simulink model "house35"  (R2022b)
settings: Solver=VariableStepAuto  StartTime=0.0  StopTime=60  RelTol=1e-3
libraries: vrlib x1
settings Model: NumberOfSteps=5  Creator=Abdiladif Hassan  LastModifiedBy=Administrator
settings OptimizationCC: ReuseModelBlockBuffer=on

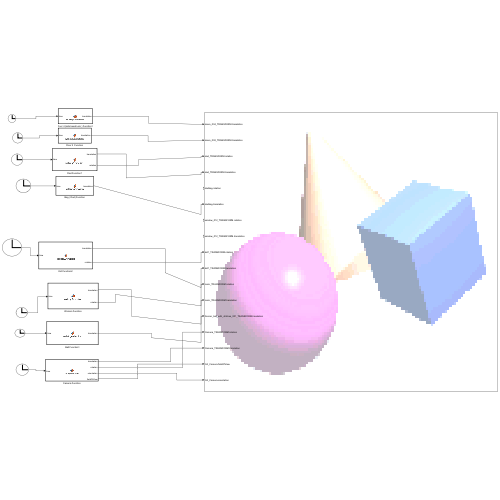
[thumbnail: Simulink's stored preview of the top-level diagram]
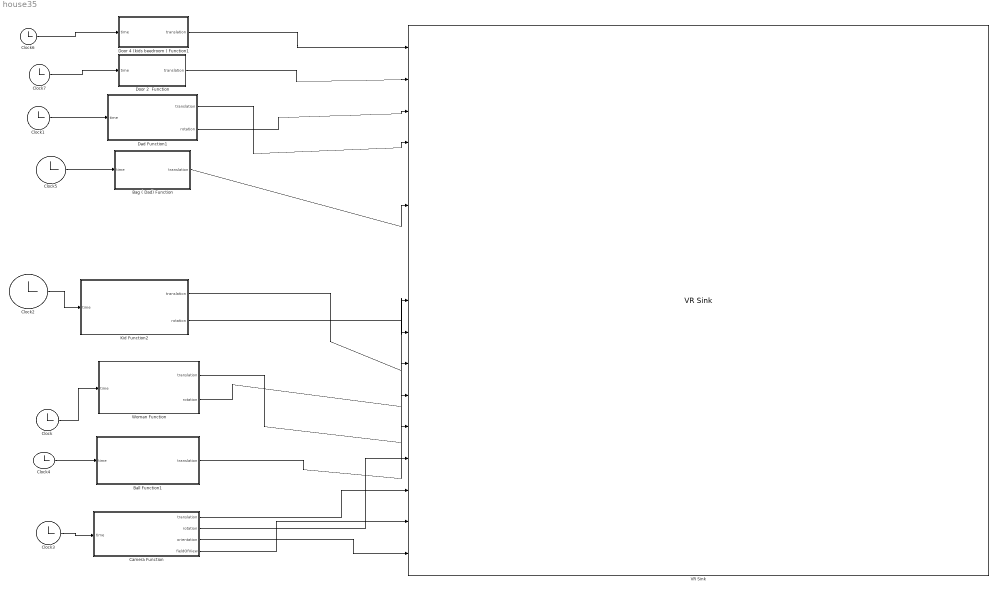
== system house35 ==
  Bag ( Dad) Function : MATLAB Function  TreatAsAtomicUnit=on
  Ball Function1 : MATLAB Function  TreatAsAtomicUnit=on
  Camera Function : MATLAB Function  TreatAsAtomicUnit=on
  Clock{,1..7} (8 alike) : Clock
  Dad Function1 : MATLAB Function  TreatAsAtomicUnit=on
  Door 2  Function : MATLAB Function  TreatAsAtomicUnit=on
  Door 4 (kids beedroom ) Function1 : MATLAB Function  TreatAsAtomicUnit=on
  Kid Function2 : MATLAB Function  TreatAsAtomicUnit=on
  VR Sink : vrlib/VR Sink  InstantiateOnLoad=on  SampleTime=0.1  ViewEnable=on  RemoteChange=off  RemoteView=off  FieldsWritten=dvere_004_TRANSFORM.translation.3.1.1.double#dvere_002_TRANSFORM.translation.3.1.1.double#dad_TRANSFORM.rotation.4.1.1.double#dad_TRANSFORM.translation.3.1.1.double#dadbag.rotation.4.1.1.double#dadbag.translation.3.1.1.double#window_012_TRANSFORM.rotation.4.1.1.double#window_012_TRANSFORM.translation.3.1.1.double#kid1_TRANSFORM.rotation.4.1.1.double#kid1_TRANSFORM.translation.3.1.1.double#mom_TRANSFORM.rotation.4.1.1.double#mom_TRANSFORM.translation.3.1.1.double#Soccer_ball_with_stitches_001_TRANSFORM.translation.3.1.1.double#Camera_TRANSFORM.rotation.4.1.1.double#Camera_TRANSFORM.translation.3.1.1.double#CA_Camera.fieldOfView.1.1.1.double#CA_Camera.orientation.4.1.1.double  WorldFileName=house35.x3d  AutoView=off  VideoDimensions=[]  AllowVariableSize=off  FigureProperties="{'Position', 'Name', 'Viewpoint', 'CameraBound', 'CameraDirection', 'CameraPosition', 'CameraUpVector', 'ZoomFactor', 'Antialiasing', 'Headlight', 'Lighting', 'NavPanel', 'Sound', 'StatusBar', 'Stereo3D', 'Stereo3DCameraOffset', 'Stereo3DHIT', 'ToolBar', 'Textures', 'Transparency', 'Triad', 'Wireframe', 'NavZones', 'NavMode', 'NavSpeed', 'CaptureFileFormat', 'CaptureFileName', 'Record2DCompressMethod', 'Record2DCompressQuality', 'Record2D', 'Record2DFileName', 'Record2DFPS'; [1.0000000000000000e+00   7.6000000000000000e+01   1.3660000000000000e+03   5.9300000000000000e+02], '', '_untitled_1', 'on', [0.0000000000000000e+00   0.0000000000000000e+00  -1.0000000000000000e+00], [0.0000000000000000e+00   0.0000000000000000e+00   0.0000000000000000e+00], [0.0000000000000000e+00   1.0000000000000000e+00   0.0000000000000000e+00], [1.0000000000000000e+00], 'on', 'on', 'on', 'halfbar', 'on', 'on', 'off', [1.0000000149011612e-01], [0.0000000000000000e+00], 'on', 'on', 'on', 'none', 'off', 'off', 'examine', 'normal', 'tif', 'C:\\Users\\Administrator\\Videos\\%f_anim_%n.tif', 'auto', [7.5000000000000000e+01], 'on', 'C:\\Users\\Administrator\\Videos\\%f_anim_%n.avi', 'auto'}"
  Woman Function : MATLAB Function  TreatAsAtomicUnit=on
  wires:
  Clock/1 -> Woman Function/1(time)
  Clock1/1 -> Dad Function1/1(time)
  Clock2/1 -> Kid Function2/1(time)
  Clock3/1 -> Camera Function/1(time)
  Clock4/1 -> Ball Function1/1(time)
  Clock5/1 -> Bag ( Dad) Function/1(time)
  Clock7/1 -> Door 2  Function/1(time)
  Clock6/1 -> Door 4 (kids beedroom ) Function1/1(time)
  Door 4 (kids beedroom ) Function1/1(translation) -> VR Sink/1
  Door 2  Function/1(translation) -> VR Sink/2
  Dad Function1/2(rotation) -> VR Sink/3
  Dad Function1/1(translation) -> VR Sink/4
  Bag ( Dad) Function/1(translation) -> VR Sink/6
  Kid Function2/2(rotation) -> VR Sink/9
  Kid Function2/1(translation) -> VR Sink/10
  Woman Function/2(rotation) -> VR Sink/11
  Woman Function/1(translation) -> VR Sink/12
  Ball Function1/1(translation) -> VR Sink/13
  Camera Function/2(rotation) -> VR Sink/14
  Camera Function/1(translation) -> VR Sink/15
  Camera Function/3(orientation) -> VR Sink/17
  Camera Function/4(fieldOfView) -> VR Sink/16

== matlab function house35/Dad Function1 ==
  data: time input; translation output; rotation output
function [translation, rotation] = walkingAnimation(time)
    % Initial position
    initial_translation = [-2.9294, 0.054634, -9.637];
    initial_rotation = [-0.31548, 0.63089, 0.70884, 2.5312];

    %%%%%%%%%%%%%%%%%%%%%%%%%%%%%%%%%%%%%%%%%%%%%%%%%%%%%%%%%%%%%%%%%
    right_rotation = [-0.99444, -0.085186, -0.061846, 1.6469];
    left_rotation = [-0.043653, 0.69547, 0.71722, 2.9948];
    back_rotation = [-0.52633, -0.56495, -0.63546, 2.2025];
    %%%%%%%%%%%%%%%%%%%%%%%%%%%%%%%%%%%%%%%%%%%%%%%%%%%%%%%%%%%%%%%%%
    
    
    % Initialize translation and rotation values
    translation = initial_translation;
    rotation = initial_rotation;
    
    % Move to house
    if time <= 5.5
        translation(1) = initial_translation(1) + 0.8 * time;
        rotation = initial_rotation;

    % get up to the staire and into the house
    elseif time >= 5.5 && time <= 15
        rotation =  right_rotation;

        translation(1) = (initial_translation(1) + 5.5) - (0.1 * time);
        translation(2) = initial_translation(2) + 0.4;
        translation(3) = initial_translation(3) + 0.45 * time;
    
     % turn after bag placement
    elseif time >=15 && time<=16
        % no walking
        translation(1) = (initial_translation(1) + 5.5) - (0.1 * 15);
        translation(2) = initial_translation(2) + 0.4;
        translation(3) = initial_translation(3) + (0.45 * 15) - (0.01 * time);

        rotation =  left_rotation;

        %get out of the room
    elseif time >=16 && time <=21
        translation(1) = (initial_translation(1) + 5.5) - (0.1 * 15) + 0.2 * time;
        translation(2) = initial_translation(2) + 0.4;
        translation(3) = initial_translation(3) + (0.45 * 15) - (0.1 * time); % redo the  (0.01 * time)

        rotation =  left_rotation;
     
     %walk to the  main entrance ( call the kid inside)
     elseif time >=21 && time <=23
        translation(1) = (initial_translation(1) + 5.5) - (0.1 * 15) + (0.1 * 21);
        translation(2) = initial_translation(2) + 0.4;
        translation(3) = initial_translation(3) + (0.45 * 15) - (0.1 * 21) + (0.1 * time);

        rotation =  right_rotation;

    % walk to the entrance (speed)
     elseif time >=23 && time <=32
        translation(1) = (initial_translation(1) + 5.5) - (0.1 * 15) + (0.1 * 21);
        translation(2) = initial_translation(2) + 0.4;
        translation(3) = initial_translation(3) + (0.45 * 15) - (0.1 * 21) + (0.3 * time);

        rotation =  right_rotation;

        %stop at the table
    elseif time >=32 && time<=60
        translation(1) = (initial_translation(1) + 5.5) - (0.1 * 15) + (0.1 * 21);
        translation(2) = initial_translation(2) + 0.4;
        translation(3) = initial_translation(3) + (0.45 * 15) - (0.1 * 21) + (0.3 * 32);

        rotation =  left_rotation;
    end
end

== matlab function house35/Woman Function ==
  data: time input; translation output; rotation output
function [translation, rotation] = walkingAnimation(time)
    % Initial position
    initial_translation = [-3.2584, 0.13427, -7.8401];
    initial_rotation = [-0.64928, 0.57913, 0.493, 2.0828];

    right_rotation = [-0.99444, -0.085186, -0.061846, 1.6469]; %woman
    left_rotation = [-0.043653, 0.69547, 0.71722, 2.9948]; %kid
    back_rotation = [-0.52633, -0.56495, -0.63546, 2.2025];
    
    % Initialize translation and rotation values
    translation = initial_translation;
    rotation = initial_rotation;
    
    %walk to the house
    if time <= 8
        translation(1) = initial_translation(1) + 0.93 * time; 
        rotation = initial_rotation;
      
    elseif time >= 8 && time <=12
        %rotation = [-0.64928, 0.57913, 0.493, 2.0828];
        rotation = right_rotation;
        translation(1) = translation(1) + 8;
        translation(2) = translation(2) + 0.25;
       
       
        translation(3) = translation(3) + 1.5*(time-8);

        %rotate to enter the house
    elseif time >= 12 && time <=15
        rotation =  right_rotation;

        %Keep walking
        translation(3) = initial_translation(3) + 0.8 * time;
        translation(1) = initial_translation(1) + 0.93 * 7.5;
        translation(2) = initial_translation(2) + 0.4;

        % stop at the table
    elseif time >= 15 && time <=60
        rotation =  back_rotation;
 
        %Keep walking
        translation(3) = initial_translation(3) + 0.8 * 14.5; % adjust from 15 for good placement
        translation(1) = initial_translation(1) + 0.93 * 7.5; % adjust from 8 for good placement
        translation(2) = initial_translation(2) + 0.4;

    end
end

== matlab function house35/Kid Function2 ==
  data: time input; translation output; rotation output
function [translation, rotation] = walkingAnimation(time)
% Initial position
initial_translation = [-3.20238, 0.082384, -11.6038];
initial_rotation = [-0.60466, 0.5304, 0.59419,1.879];

right_rotation = [-0.99444, -0.085186, -0.061846, 1.6469]; %woman
left_rotation = [-0.043653, 0.69547, 0.71722, 2.9948]; %kid
back_rotation = [-0.52633, -0.56495, -0.63546, 2.2025];%woman

% Initialize translation and rotation values
translation = initial_translation;
rotation = initial_rotation;

% kid goes to the ball
if time <= 8
    translation(1) = initial_translation(1) + 0.7 * time;
    rotation = initial_rotation;

    %kid is next to the ball
elseif time >=8 && time <=21
    translation(2) = initial_translation(2) - (0.05 * 1 * (1 - 2 * rem(time, 2)));
    translation(1) = (initial_translation(1) + 0.7 * 8) + ((0.05 * 1 * (1 - 2 * rem(time, 2))));
    rotation =  back_rotation;


    %walk to the house
elseif time>=21 && time<=22
    translation(1) = initial_translation(1) + 0.7 * 8;
    translation(3) = initial_translation(3) + 0.1 * time;

    rotation = right_rotation;

    %get up in the staires and walk into the house
elseif time>=22 && time<=35
    translation(1) = initial_translation(1) + 0.7 * 8 + 2; % + 2 to get strait into the main entrance
    

    translation(2) = initial_translation(2) + 0.4;
    translation(3) = initial_translation(3) + (0.1 * 22) + 0.3 * time;

    rotation = right_rotation;

  % walk to the table
elseif time >=35 && time <=37
    translation(1) = initial_translation(1) + 0.7 * 8;
    translation(2) = initial_translation(2) + 0.4;
    translation(3) = initial_translation(3) + (0.1 * 22) + (0.3 * 35) + (0.07 * time);

    rotation = right_rotation;

%stop at the talbe
elseif time>=37 && time<=50
    translation(1) = initial_translation(1) + 0.7 * 8;
    translation(2) = initial_translation(2) + 0.4;
    translation(3) = initial_translation(3) + (0.1 * 22) + (0.3 * 35) + (0.07 * 37);

    rotation = initial_rotation;

 %turn left to go to the bedroom
elseif time>=50 && time<=51
    translation(1) = initial_translation(1) + 0.7 * 8;
    translation(2) = initial_translation(2) + 0.4;
    translation(3) = initial_translation(3) + (0.1 * 22) + (0.3 * 35) + (0.07 * 37) - (0.01 * time);

    rotation = left_rotation;

 % Walk to go to the bedroom
elseif time>=51 && time<=54
    translation(1) = initial_translation(1) + 0.7 * 8;
    translation(2) = initial_translation(2) + 0.4;
    translation(3) = initial_translation(3) + (0.1 * 22) + (0.3 * 35) + (0.07 * 37) - (0.08 * time);

    rotation = left_rotation;


%next to door 2
elseif time>= 54 && time <=57
    translation(1) = initial_translation(1) + 0.7 * 8 -1; % -1 to get closer to the door
    translation(2) = initial_translation(2) + 0.4;
    translation(3) = initial_translation(3) + (0.1 * 22) + (0.3 * 35) + (0.07 * 37) - (0.08 * 54);

    rotation = back_rotation;

   %get the kid into his room
elseif time >=57 && time<=58
    translation(1) = initial_translation(1) + 0.7 * 8 - 5;  % -5 to place him in his room
    translation(2) = initial_translation(2) + 0.4;
    translation(3) = initial_translation(3) + (0.1 * 22) + (0.3 * 35) + (0.07 * 37) - (0.08 * 54) - 2; % -2 to place him in his room
    rotation = back_rotation;

    %kid walks inside his room
elseif time >=58 && time<=60
    translation(1) = initial_translation(1) + 0.7 * 8 - 5 - (0.01 * time); 
    translation(2) = initial_translation(2) + 0.4;
    translation(3) = initial_translation(3) + (0.1 * 22) + (0.3 * 35) + (0.07 * 37) - (0.08 * 54) - 2  - (0.01 * time);

    rotation = back_rotation;
else
    translation(1) = initial_translation(1) + 0.7 * 8 -1;
    translation(2) = initial_translation(2) + 0.4;
    translation(3) = initial_translation(3) + (0.1 * 22) + (0.3 * 35) + (0.07 * 37) - (0.08 * 54) ;

    rotation = left_rotation;



end
end

== matlab function house35/Camera Function ==
  data: time input; translation output; rotation output; orientation output; fieldOfView output
function [translation, rotation, orientation, fieldOfView] = cameraMotion(time)
    
   %camera positions
    initial_translation = [5.48, 5.12, -15.75];
    main_beedroom = [1.59, 2.28, -4.68];
    main_entrance = [9.488, 1.8306, -3.3051];
    setting_room1 = [2.63, 2.19, -2.05];
    setting_room2 = [4.99, 2.52, 5.27];

    initial_rotation = [-0.015123, 0.99278, 0.11903, 2.8907];
    initial_orientation = [-0.43, -0.89, 0.14, 0];
    initial_fielOfView = 1.466;
    %main_entrance_rotation = [0.01976, 0.99972, -0.013307, 1.1857];
    main_entrance_rotation = [-0.31976, 0.99972, 0.313307, 1.1857];
    right_rotation = [-0.99444, -0.085186, -0.061846, 1.6469];
    left_rotation = [-0.043653, 0.69547, 0.71722, 2.9948];
    back_rotation = [-0.52633, -0.56495, -0.63546, 2.2025];
    
    
    % Initialize translation and rotation values
    translation =initial_translation;
    rotation = initial_rotation;
    orientation = initial_orientation;
    fieldOfView = initial_fielOfView;

    
% start camera
    if time <= 5.5
        translation =initial_translation;
        rotation = initial_rotation;
        
        %translation = [-2.94, 2.86, -5.03];
        %rotation = [-0.31976, 0.99972, 0.313307, 3.1857] ;
    elseif time >=5.5 && time <=13
         translation(1) =initial_translation(1)+2;
        rotation = initial_rotation;
        orientation = [-0.43, -0.89, 0.14, 1];


 %main beedroom
    elseif time >= 13 && time <= 16
        translation = main_beedroom;
        rotation = initial_rotation;
    
    %main entrance

    elseif time >=16 && time <=22
         orientation = [-0.43, -0.89, 0.14, 1];

    elseif time>=22 && time <=26
        translation = main_entrance;
        rotation = main_entrance_rotation;
    
      % settting room camera
    elseif time>=26 && time <=35
        translation = setting_room1;
        rotation = initial_rotation;

    elseif time >=35 && time <=37
        fieldOfView = 0.3;


          % settting room camera 2 
    elseif time>=37 && time <=40
        translation = setting_room2;
        rotation = main_entrance_rotation;

        %%%%%%%%%%%% Switch the two cameras in the setting room %%%%%%%
   
    % Switch Camera settting room camera 1
    elseif time>=40 && time <=43
        translation = setting_room1;
        rotation = initial_rotation;
    
          % Switch to settting room camera 2 
    elseif time>=43 && time <=46
        translation = setting_room2;
        rotation = main_entrance_rotation;

       % Switch Camera settting room camera 1
    elseif time>=46 && time <=49
        translation = setting_room1;
        rotation = initial_rotation;
    
          % Switch to settting room camera 2 
    elseif time>=49 && time <=52
        translation = setting_room2;
        rotation = main_entrance_rotation;
   
    % Switch Camera settting room camera 1
    elseif time>=52 && time <=58
        translation = setting_room1;
        rotation = initial_rotation;

        %kids beedroom
    elseif time >=58 && time<=60
        translation = [-2.94, 2.86, -5.03];
        rotation = [-0.31976, 0.99972, 0.313307, 3.1857] ;
   
    else
        translation = setting_room2;
        rotation = main_entrance_rotation;     
    end
end

== matlab function house35/Ball Function1 ==
  data: time input; translation output
function translation = walkingAnimation(time)
    % Initial position
    initial_translation = [2.09762, 0.082384, -11.6038];
    initial_rotation = [0, 0.70711, 0.70711, 3.1416];
    
    translation = initial_translation;
    rotation = initial_rotation;
    
  
    if time >=9 && time <=20
        %translation(2) = translation(2) - 0.1 * time;
         translation(2) = initial_translation(2) - (0.1 * 4 * (1 - 2 * rem(time, 2)));
    end
end

== matlab function house35/Bag ( Dad) Function ==
  data: time input; translation output
function translation  = walkingAnimation(time)
    % Initial position
    initial_translation = [0, 0, 0];
    %initial_rotation = [0, 0, 1, 0];

    %%%%%%%%%%%%%%%%%%%%%%%%%%%%%%%%%%%%%%%%%%%%%%%%%%%%%%%%%%%%%%%%%
    right_rotation = [-0.99444, -0.085186, -0.061846, 1.6469];
    left_rotation = [-0.043653, 0.69547, 0.71722, 2.9948];
    back_rotation = [-0.52633, -0.56495, -0.63546, 2.2025];
    %%%%%%%%%%%%%%%%%%%%%%%%%%%%%%%%%%%%%%%%%%%%%%%%%%%%%%%%%%%%%%%%%
    
    
    % Initialize translation and rotation values
    translation = initial_translation;
    %rotation = initial_rotation;
    

    % get up to the staire and into the house
    if time >= 15
        translation = [-1.0044, -20.1853, 0.7736];
    end
end

== matlab function house35/Door 2  Function ==
  data: time input; translation output
function translation  = walkingAnimation(time)
    translation = [-0.92003, -1.2222, 0.43461];
    %walk to the house
    if time >= 55
        translation(2) = translation(2) + 20; 
    end
end

== matlab function house35/Door 4 (kids beedroom ) Function1 ==
  data: time input; translation output
function translation  = walkingAnimation(time)
    translation = [2.475, -2.04, 0.43461];
    %walk to the house
    if time >= 55
        translation(2) = translation(2) + 20; 
    end
end
